simulink model "sensorMCUSlugsMKII_ren"  (Simulink 6.6)
settings: Solver=FixedStepDiscrete  StartTime=0.0  StopTime=10.0  FixedStep=0.01  RelTol=1e-3
InitFcn:
  | mcuInit
values from neighbouring files (symbols this model uses):
  accBiasRateLimit = 2*(.014844)/300*apSampleTime    [mcuInit.m]
  accelXCutTemp = 350.0    (= 350)    [mcuInit.m]
  axTGain1 = -0.0332796    [mcuInit.m]
  axTGain2 = 0.0543519    [mcuInit.m]
  axTMean1 = 68.41    [mcuInit.m]
  axTMean2 = 500.7    [mcuInit.m]
  barAdjust = -6    [mcuInit.m]
  baroCutoff = 0.38/(2*pi)    (= 0.0604788783749)    [mcuInit.m]
  baroCutTemp = -50.0    (= -50)    [mcuInit.m]
  baroOffset = P(2)    [mcuInit.m]
  baroScale = P(1)    [mcuInit.m]
  barTGain1 = -0.0102663    [mcuInit.m]
  barTGain2 = 0.0207608    [mcuInit.m]
  barTMean1 = -161.3    [mcuInit.m]
  barTMean2 = 347.23    [mcuInit.m]
  baseTemp = 288.215    [mcuInit.m]
  cubeAccelGain = (2.522e-3)*9.815    (= 0.02475343)    [mcuInit.m]
  cubeGyroGain = .07326*pi/180    (= 0.00127862821001)    [mcuInit.m]
  gyroBiasRateLimit = 2*(.006393)/500*apSampleTime    [mcuInit.m]
  lapseRate = -0.00198122    [mcuInit.m]
  lowRateSensorCutoff = 0.02    [mcuInit.m]
  magMeanTemp = [162.42 162.42 162.42]    [mcuInit.m]
  magOffset = 0    [mcuInit.m]
  magScale = 0.3418    [mcuInit.m]
  magTempK = [.0057 -.0423 .0426]    [mcuInit.m]
  mainSensorCutoff = 10    [mcuInit.m]
  maxDynPressure = 3000    [mcuInit.m]
  pitAdjust = -41    [mcuInit.m]
  pitCutTemp = -130.0    (= -130)    [mcuInit.m]
  pitotOffset = -1083.881038056753    (= -1083.88103806)    [mcuInit.m]
  pitotScale = 1.213292590242    (= 1.21329259024)    [mcuInit.m]
  pitTGain1 = -0.0552923    [mcuInit.m]
  pitTGain2 = -0.0950433    [mcuInit.m]
  pitTMean1 = -202.93    [mcuInit.m]
  pitTMean2 = 293.053    [mcuInit.m]
  powerOffset = P(2)    [mcuInit.m]
  powerScale = P(1)    [mcuInit.m]
  pressureSensorCutoff = 5    [mcuInit.m]
  T = 0.01    [initGPS.m]    (also in mcuInit.m)
  tempOffset = P(2)    [mcuInit.m]
  tempScale = P(1)    [mcuInit.m]
  vzCutoff = 2    [mcuInit.m]
  xCutoff = 10    [mcuInit.m]
  yCutoff = 10    [mcuInit.m]
  zCutoff = 0.2    [mcuInit.m]
undefined symbols (not defined in the file or in its folder): apSampleTime, baseHeight, DiscIntNeverNeededParam, gaind, getCubeData, getGpsMainData, getMag, GS_location, hil_getEuler, hil_getRates, hil_getRawRead, hil_getVned, hil_getXYZ, hilRead, logData, param_acc, param_mag, polesd, protParseDecode, q_quat, sensorMCUInit, spiSend, u1, u2, updateAirData, updateAttitude, updateBias, updateDiagnosticFl, updateDiagnosticSh, updateLoadData, updatePilotConsole, updatePosition, updateRawADCData, updateTimeStamp, Vb_0, y1, zerosd
libraries: dsPICdrivers x45, simulink x13, aerolibutil x4, dspmtrx3 x2, aerolibconvert2 x2
(part 1 of 4)
settings Model: Creator=ASL_Lab  LastModifiedBy=Administrator  BufferReuse=off  ProdHWDeviceType=16-bit Generic
settings OptimizationCC: BlockReduction=off  InlineParams=on  OptimizeBlockIOStorage=off  BufferReuse=off  ExpressionFolding=off  LocalBlockOutputs=off  EfficientFloat2IntCast=on  OptimizeModelRefInitCode=on  LifeSpan=1
settings HardwareCC: ProdBitPerInt=16  ProdEndianess=LittleEndian  ProdWordSize=16  ProdHWDeviceType=16-bit Generic  TargetHWDeviceType=32-bit Generic
settings RTWCC: SystemTargetFile=dspic.tlc  TemplateMakefile=dspic_pic30_gcc.tmf  PostCodeGenCommand=dsPIC_Compile()  Description=Embedded Target for Microchip dsPIC (real-time)  GenerateReport=on  ProcessScript=dspic_make_rtw_hook  CustomHeaderCode="#include \"apDefinitions.h\""  IncludeHyperlinkInReport=on  LaunchReport=on
settings RTWCC: CustomSource=|
  | clib\circBuffer.c
  | clib\sbrk.c
  | clib\gps.c
  | clib\dataLogger.c
  | clib\interProcCommMaster.c
  | clib\conversions.c
  | clib\apUtils.c
  | clib\protDecoder.c
  | clib\DEE.c
  | clib\DEES.s
  | clib\magneto.c
  | clib\adisCube.c
settings CodeAppCC: IgnoreCustomStorageClasses=off
settings STFCustomTargetCC: TargetFcnLib=ansi_tfl_tmw.mat  GenFloatMathFcnCalls=ANSI_C  ModelReferenceCompliant=off  IncludeMdlTerminateFcn=off  CombineOutputUpdateFcns=on  SuppressErrorStatus=on  ERTCustomFileBanners=on  SupportContinuousTime=off  SupportNonInlinedSFcns=off  SystemTargetFile=dspic.tlc
settings ERTTargetCC: TargetFcnLib=ansi_tfl_tmw.mat  GenFloatMathFcnCalls=ANSI_C  ModelReferenceCompliant=off  IncludeMdlTerminateFcn=off  SuppressErrorStatus=on  ModelStepFunctionPrototypeControlCompliant=off  ExtModeMexFile=noextcomm  InlinedParameterPlacement=NonHierarchical  ERTSrcFileBannerTemplate=dsPIC_code_template.cgt  ERTHdrFileBannerTemplate=dsPIC_code_template.cgt  ERTDataSrcFileTemplate=dsPIC_code_template.cgt  ERTDataHdrFileTemplate=dsPIC_code_template.cgt  ERTCustomFileTemplate=dsPIC_main.tlc
settings CustomProperty: DataType=string  Value=C:\PROGRA~1\MATLAB\R2007a\rtw\bin\win32\gmake

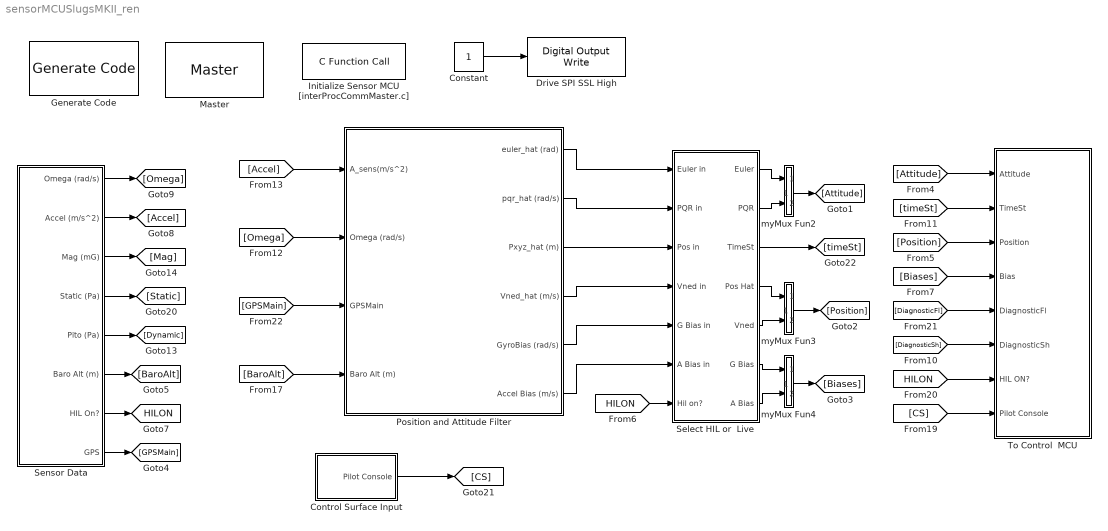
== system sensorMCUSlugsMKII_ren ==
  Constant : Constant  OutDataTypeMode=boolean
  Control Surface Input : Subsystem
  Drive SPI SSL High : dsPICdrivers/Digital I//O/Digital Output Write  Tag=dsPIC_Digital_Output  Priority=5  PORT=B  Pin=[ 2]  Simultaneous=off  OrderingInOutPopup=None
  Generate Code : dsPICdrivers/Simulink Configuration/Generate Code
  Initialize Sensor MCU [interProcCommMaster.c] : dsPICdrivers/OTHERS/C Function Call  Tag=dsPIC_dsPIC_CFunctionCall  fctName='sensorMCUInit'  INPUT_SIZE=1  INPUT1=--  INPUT2=--  INPUT3=--  OUTPUT_SIZE=1  OUTPUT1=--  SampleTime=inf  InputType=[ ]  OutputType=[ ]  FctDeclaration=extern void sensorMCUInit();  FctCall=sensorMCUInit();  OrderingInOutPopup=None
  Master : dsPICdrivers/Master  Tag=dsPIC_MASTER  Priority=1  TimeStepType=Timer1  picType=33fJ256MC710  fcy=40000000  Quartz_33f=12e6  PLLActive_33f=on  fcyDesired_33f=40e6  tmr1="[8  49999  0]"  tmr1Info="Time Step : 0.01  ;   Error : 0%  PR1=49999"  tmr2345="[8  0  0  0  0  0  0  0]"  tmr2345cfg=[-1 -1 -1 -1 -1 -1 -1 -1]  IOautoConf=on  typePort="[ 0   0   0   0   0   0   0   0   0   0   0   0   0   0   9   0   0   0  10   0   0   0   0   0   8   8   8   8   0   0   0   0   0   0   0   0   0   0   0   0   0   0   0   0   0   0   0   0   0   0   9   0   0   0   0   0   0   6   6   6   6   0   0   6   0   0   0   0   0   0   0   0   0   0   0   0   0   0   0   0   0   0   0   0   0   0   0   0   0   0   0   0   0   0   0   0   0   0   0   0   0   0   0   0   0   0   0   0   0   0   0   0 ]"  TRIS="[ 65535  65531  65535  65535  65535  65535  65535 ]"  ADPCFG=4  MasterBusyPort=None  MasterOverloadPort=None  FOSC=External Clock  ClockSwitchMonitor=Both disabled  TempProtection_33f=TEMP_ON  FPBOR=<empty>  PWRT=64ms  MCLR=<empty>  PowerSave=off  OverrideFcy=off  NewFcy=1e6  PR2345="[65535  65535  65535  65535  65535  65535  65535  65535]"
  Position and Attitude Filter : Subsystem
  Select HIL or  Live : Subsystem
  Sensor Data : Subsystem
  To Control  MCU : Subsystem
  myMux Fun2 : Stateflow chart
  myMux Fun3 : Stateflow chart
  myMux Fun4 : Stateflow chart
  tag scope: HILON=global
  wires:
  Constant/1 -> Drive SPI SSL High/1
  myMux Fun2/1(y) -> [Attitude]
  myMux Fun3/1(y) -> [Position]
  myMux Fun4/1(y) -> [Biases]
  Control Surface Input/1(Pilot Console) -> [CS]
  [Position] -> To Control  MCU/3(Position)
  [Biases] -> To Control  MCU/4(Bias)
  [DiagnosticFl] -> To Control  MCU/5(DiagnosticFl)
  [HILON] -> To Control  MCU/7(HIL ON?)
  [CS] -> To Control  MCU/8(Pilot Console)
  [Attitude] -> To Control  MCU/1(Attitude)
  Select HIL or  Live/1(Euler) -> myMux Fun2/1(u1)
  Select HIL or  Live/2(PQR) -> myMux Fun2/2(u2)
  Select HIL or  Live/3(TimeSt) -> [timeSt]
  Select HIL or  Live/4(Pos Hat) -> myMux Fun3/1(u1)
  Select HIL or  Live/5(Vned) -> myMux Fun3/2(u2)
  Select HIL or  Live/6(G Bias) -> myMux Fun4/1(u1)
  Select HIL or  Live/7(A Bias) -> myMux Fun4/2(u2)
  [DiagnosticSh] -> To Control  MCU/6(DiagnosticSh)
  [timeSt] -> To Control  MCU/2(TimeSt)
  Sensor Data/2(Accel (m/s^2)) -> [Accel]
  Sensor Data/1(Omega (rad/s)) -> [Omega]
  Sensor Data/3(Mag (mG)) -> [Mag]
  Sensor Data/4(Static (Pa)) -> [Static]
  Sensor Data/5(Pito (Pa)) -> [Dynamic]
  Sensor Data/6(Baro Alt (m)) -> [BaroAlt]
  Sensor Data/7(HIL On?) -> [HILON]
  Sensor Data/8(GPS) -> [GPSMain]
  [HILON] -> Select HIL or  Live/7(Hil on?)
  [Omega] -> Position and Attitude Filter/2(Omega (rad/s))
  [Accel] -> Position and Attitude Filter/1(A_sens(m/s^2))
  Position and Attitude Filter/1(euler_hat (rad)) -> Select HIL or  Live/1(Euler in)
  Position and Attitude Filter/2(pqr_hat (rad/s)) -> Select HIL or  Live/2(PQR in)
  Position and Attitude Filter/3(Pxyz_hat (m)) -> Select HIL or  Live/3(Pos in)
  Position and Attitude Filter/4(Vned_hat (m/s)) -> Select HIL or  Live/4(Vned in)
  Position and Attitude Filter/5(GyroBias (rad/s)) -> Select HIL or  Live/5(G Bias in)
  Position and Attitude Filter/6(Accel Bias (m/s)) -> Select HIL or  Live/6(A Bias in)
  [GPSMain] -> Position and Attitude Filter/3(GPSMain)
  [BaroAlt] -> Position and Attitude Filter/4(Baro Alt (m))

== system sensorMCUSlugsMKII_ren/Control Surface Input ==
  Input Capture : dsPICdrivers/Peripheral I//O/Input Capture  Tag=dsPIC_PWM_IC  Priority=5  IntPriority=6  Channel=[ 2 3 4 5 8]  Channel_UP_Down_Periode="[1  1  1  1  1]"  MaxChannel="[0.0025      0.0025      0.0025      0.0025      0.0025]"  SafeMarge="[10  10  10  10  10]"  MaxName=' IC2max , IC3max , IC4max , IC5max , IC8max '  Precision="[13.7469      13.7469      13.7469      13.7469      13.7469]"  Timer="[2  2  2  2  2]"  ChangeDetected="[0  0  0  0  0]"  ChangeDetectedPortRef=3  SampleTime=.01  Status=OK
  myMux Fun5 : Stateflow chart
  Pilot Console : Outport
  wires:
  myMux Fun5/1(y) -> Pilot Console/1
  Input Capture/1 -> myMux Fun5/1(u1)
  Input Capture/2 -> myMux Fun5/2(u2)
  Input Capture/3 -> myMux Fun5/3(u3)
  Input Capture/4 -> myMux Fun5/4(u4)
  Input Capture/5 -> myMux Fun5/5(u5)

== system sensorMCUSlugsMKII_ren/Position and Attitude Filter ==
  A_sens(m/s^2) : Inport
  Omega (rad/s) : Inport  Port=2
  GPSMain : Inport  Port=3
  Baro Alt (m) : Inport  Port=4
  Attitude Complimentary Filter COG : Subsystem
  COG.SOG2V : Subsystem
  Compute GS Location : Subsystem
  Constant : Constant  Value=GS_location  OutDataTypeMode=single
  Demux : Demux  Outputs=5
  GPS Update : Subsystem  mask{T=0.01}
      mask prompts: T "Sample Time"
  Geod2LTP1 : Subsystem
      mask Description:
      | This block provides transformation of the Geodetic coordinates
      | to the LTP coorinate system. The block uses two consecutive transformations
      | (Geodetic -> ECEF ->LTP).
      | Geodetic coordinates of the LTP origin should also be predetermined.
      mask Help: Oops!
      mask Display: plot(0,0,100,100,[45,40,35,40,40],[85,95,85,95,40],[85,95,85,95,40],[35,40,45,40,40],[60,40,10,20,10,14],[70,40,10,13,10,20],[56,45],[70,70],[60,60],[50,60],[60,60],[30,40],[50,60],[20,20],[30,40],[20,20],[45,55],[35,25],[75,65],[35,25])
  Position Filter : Subsystem
  "[1 1 -1]" : Gain  Gain=[1 1 -1]
  euler_hat (rad) : Outport
  pqr_hat (rad/s) : Outport  Port=2
  Pxyz_hat (m) : Outport  Port=3
  Vned_hat (m/s) : Outport  Port=4
  GyroBias (rad/s) : Outport  Port=5
  Accel Bias (m/s) : Outport  Port=6
  wires:
  Position Filter/1(Vxyd_hat) -> Vned_hat (m/s)/1, Attitude Complimentary Filter COG/4(Vxyd_hat)
  Position Filter/2(Pxyd_hat) -> Pxyz_hat (m)/1
  Position Filter/3(acc_bias) -> Accel Bias (m/s)/1, Attitude Complimentary Filter COG/5(acc_bias)
  Geod2LTP1/1("NEU, m") -> GPS Update/1(XYZ), "[1 1 -1]"/1
  Attitude Complimentary Filter COG/4(RL2B) -> Position Filter/3(RLT2B)
  Attitude Complimentary Filter COG/1(euler_hat) -> euler_hat (rad)/1
  Attitude Complimentary Filter COG/2(pqr_hat) -> pqr_hat (rad/s)/1
  Attitude Complimentary Filter COG/3(Gyro Bias) -> GyroBias (rad/s)/1
  GPSMain/1 -> Demux/1
  Constant/1 -> Compute GS Location/1(GS Location)
  Demux/1 -> Geod2LTP1/3("Lat, deg(GPS)")
  Demux/2 -> Geod2LTP1/4("Lon, deg(GPS)")
  Demux/3 -> Geod2LTP1/5(Hight,m(GPS))
  Compute GS Location/2(R_in) -> Geod2LTP1/2(GS ECEF)
  Compute GS Location/1("Lat, Lon") -> Geod2LTP1/1(GS Lat,Lon)
  GPS Update/1(Update?) -> Position Filter/6(NewGPS)
  A_sens(m/s^2)/1 -> Attitude Complimentary Filter COG/1(A_sens)
  Omega (rad/s)/1 -> Attitude Complimentary Filter COG/3(Gyros)
  "[1 1 -1]"/1 -> Position Filter/2(GPS_XYD)
  [XY_Orient] -> Attitude Complimentary Filter COG/2(XY Orient)
  Baro Alt (m)/1 -> Position Filter/1(Baro Alt)
  Demux/4 -> COG.SOG2V/1(COG_D)
  Demux/5 -> COG.SOG2V/2(SOG), Position Filter/7(SOG)
  COG.SOG2V/1(Vnorth) -> Position Filter/4(Vnorth)
  COG.SOG2V/2(Veast) -> Position Filter/5(Veast)
  COG.SOG2V/3(XY Orient) -> [XY_Orient]

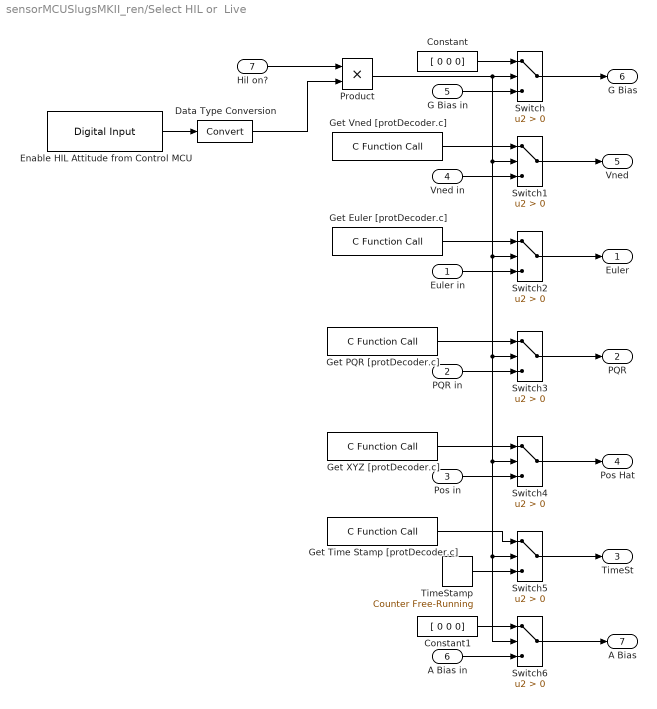
== system sensorMCUSlugsMKII_ren/Select HIL or  Live ==
  Euler in : Inport
  PQR in : Inport  Port=2
  Pos in : Inport  Port=3
  Vned in : Inport  Port=4
  G Bias in : Inport  Port=5
  A Bias in : Inport  Port=6
  Hil on? : Inport  Port=7
  Constant : Constant  Value=[ 0 0 0]  OutDataTypeMode=single
  Constant1 : Constant  Value=[ 0 0 0]  OutDataTypeMode=single
  Data Type Conversion : DataTypeConversion  OutDataTypeMode=uint8
  Enable HIL Attitude from Control MCU : dsPICdrivers/Digital I//O/Digital Input  Tag=dsPIC_Digital_Input  PORT=A  Pin=[14]  SampleTime=.01  OrderingInOutPopup=None
  Get Euler [protDecoder.c] : dsPICdrivers/OTHERS/C Function Call  Tag=dsPIC_dsPIC_CFunctionCall  fctName='hil_getEuler'  INPUT_SIZE=1  INPUT1=--  INPUT2=--  INPUT3=--  OUTPUT_SIZE=3  OUTPUT1=real32  SampleTime=.01  InputType=[ ]  OutputType=[ 7 ]  FctDeclaration=extern void hil_getEuler(real32_T* y1);  FctCall=hil_getEuler(*%y1);  OrderingInOutPopup=None
  Get PQR [protDecoder.c] : dsPICdrivers/OTHERS/C Function Call  Tag=dsPIC_dsPIC_CFunctionCall  fctName='hil_getRates'  INPUT_SIZE=1  INPUT1=--  INPUT2=--  INPUT3=--  OUTPUT_SIZE=3  OUTPUT1=real32  SampleTime=.01  InputType=[ ]  OutputType=[ 7 ]  FctDeclaration=extern void hil_getRates(real32_T* y1);  FctCall=hil_getRates(*%y1);  OrderingInOutPopup=None
  Get Time Stamp [protDecoder.c] : dsPICdrivers/OTHERS/C Function Call  Tag=dsPIC_dsPIC_CFunctionCall  fctName='hil_getTs'  INPUT_SIZE=1  INPUT1=--  INPUT2=--  INPUT3=--  OUTPUT_SIZE=1  OUTPUT1=uint16  SampleTime=.01  InputType=[ ]  OutputType=[ 4 ]  FctDeclaration=extern uint16_T hil_getTs();  FctCall=%y1 = hil_getTs();  OrderingInOutPopup=None
  Get Vned [protDecoder.c] : dsPICdrivers/OTHERS/C Function Call  Tag=dsPIC_dsPIC_CFunctionCall  fctName='hil_getVned'  INPUT_SIZE=1  INPUT1=--  INPUT2=--  INPUT3=--  OUTPUT_SIZE=3  OUTPUT1=real32  SampleTime=.01  InputType=[ ]  OutputType=[ 7 ]  FctDeclaration=extern void hil_getVned(real32_T* y1);  FctCall=hil_getVned(*%y1);  OrderingInOutPopup=None
  Get XYZ [protDecoder.c] : dsPICdrivers/OTHERS/C Function Call  Tag=dsPIC_dsPIC_CFunctionCall  fctName='hil_getXYZ'  INPUT_SIZE=1  INPUT1=--  INPUT2=--  INPUT3=--  OUTPUT_SIZE=3  OUTPUT1=real32  SampleTime=.01  InputType=[ ]  OutputType=[ 7 ]  FctDeclaration=extern void hil_getXYZ(real32_T* y1);  FctCall=hil_getXYZ(*%y1);  OrderingInOutPopup=None
  Product : Product  OutDataTypeMode=uint8  RndMeth=Zero
  Switch{,1..6} (7 alike) : Switch  Criteria=u2 > Threshold
  TimeStamp : simulink/Sources/Counter Free-Running  SystemSampleTime=-1  NumBits=16  tsamp=.01
  Euler : Outport
  PQR : Outport  Port=2
  TimeSt : Outport  Port=3
  Pos Hat : Outport  Port=4
  Vned : Outport  Port=5
  G Bias : Outport  Port=6
  A Bias : Outport  Port=7
  wires:
  Switch/1 -> G Bias/1
  Constant/1 -> Switch/1
  Product/1 -> Switch/2, Switch1/2, Switch2/2, Switch3/2, Switch4/2, Switch5/2, Switch6/2
  G Bias in/1 -> Switch/3
  Switch1/1 -> Vned/1
  Get Vned [protDecoder.c]/1 -> Switch1/1
  Vned in/1 -> Switch1/3
  Get Euler [protDecoder.c]/1 -> Switch2/1
  Euler in/1 -> Switch2/3
  Switch2/1 -> Euler/1
  Get PQR [protDecoder.c]/1 -> Switch3/1
  PQR in/1 -> Switch3/3
  Switch3/1 -> PQR/1
  Get XYZ [protDecoder.c]/1 -> Switch4/1
  Pos in/1 -> Switch4/3
  Switch4/1 -> Pos Hat/1
  TimeStamp/1 -> Switch5/3
  Get Time Stamp [protDecoder.c]/1 -> Switch5/1
  Enable HIL Attitude from Control MCU/1 -> Data Type Conversion/1
  Hil on?/1 -> Product/1
  Data Type Conversion/1 -> Product/2
  Switch5/1 -> TimeSt/1
  Switch6/1 -> A Bias/1
  Constant1/1 -> Switch6/1
  A Bias in/1 -> Switch6/3

== system sensorMCUSlugsMKII_ren/Sensor Data ==
  Data Type Conversion : DataTypeConversion  OutDataTypeMode=uint8  SampleTime=0.01
  Enable HIL from  Control MCU : dsPICdrivers/Digital I//O/Digital Input  Tag=dsPIC_Digital_Input  PORT=D  Pin=[2]  SampleTime=.01  OrderingInOutPopup=None
  Raw HIL  Readings : Subsystem
  Sensor Suite : Subsystem
  Omega (rad/s) : Outport
  Accel (m/s^2) : Outport  Port=2
  Mag (mG) : Outport  Port=3
  Static (Pa) : Outport  Port=4
  Pito (Pa) : Outport  Port=5
  Baro Alt (m) : Outport  Port=6
  HIL On? : Outport  Port=7
  GPS : Outport  Port=8
  wires:
  Raw HIL  Readings/1(Raw Msg) -> Sensor Suite/2(Raw HIL)
  Enable HIL from  Control MCU/1 -> Raw HIL  Readings/Enable, Sensor Suite/1(D2), Data Type Conversion/1
  Data Type Conversion/1 -> HIL On?/1
  Sensor Suite/1(Omega (rad/s)) -> Omega (rad/s)/1
  Sensor Suite/2(Accel (m/s^2)) -> Accel (m/s^2)/1
  Sensor Suite/3(Mag (mG)) -> Mag (mG)/1
  Sensor Suite/4(Static (Pa)) -> Static (Pa)/1
  Sensor Suite/5(Pitot (Pa)) -> Pito (Pa)/1
  Sensor Suite/6(Baro Alt (m)) -> Baro Alt (m)/1
  Sensor Suite/7(GPS) -> GPS/1

== system sensorMCUSlugsMKII_ren/To Control  MCU ==
  Attitude : Inport
  TimeSt : Inport  Port=2
  Position : Inport  Port=3
  Bias : Inport  Port=4
  DiagnosticFl : Inport  Port=5
  DiagnosticSh : Inport  Port=6
  HIL ON? : Inport  Port=7
  Pilot Console : Inport  Port=8
  IPC Data : Subsystem
  Send Debug  Data to Serial Port and Prepare for SPI [dataLogger.c] : dsPICdrivers/OTHERS/C Function Call  Tag=dsPIC_dsPIC_CFunctionCall  fctName='logData'  INPUT_SIZE=1  INPUT1=uint8  INPUT2=--  INPUT3=--  OUTPUT_SIZE=104  OUTPUT1=uint8  SampleTime=-1  InputType=[ 2 ]  OutputType=[ 2 ]  FctDeclaration=extern void logData(uint8_T u1,uint8_T* y1);  FctCall=logData(%u1, *%y1);  OrderingInOutPopup=Input
  Update Biases [dataLogger.c] : dsPICdrivers/OTHERS/C Function Call  Tag=dsPIC_dsPIC_CFunctionCall  fctName='updateBias'  INPUT_SIZE=6  INPUT1=real32  INPUT2=--  INPUT3=--  OUTPUT_SIZE=1  OUTPUT1=--  SampleTime=.01  InputType=[ 7 ]  OutputType=[ ]  FctDeclaration=extern void updateBias(real32_T* u1);  FctCall=updateBias(*%u1);  OrderingInOutPopup=Input & Output
  Update Diagnostic Float [dataLogger.c] : dsPICdrivers/OTHERS/C Function Call  Tag=dsPIC_dsPIC_CFunctionCall  fctName='updateDiagnosticFl'  INPUT_SIZE=3  INPUT1=real32  INPUT2=--  INPUT3=--  OUTPUT_SIZE=1  OUTPUT1=--  SampleTime=.01  InputType=[ 7 ]  OutputType=[ ]  FctDeclaration=extern void updateDiagnosticFl(real32_T* u1);  FctCall=updateDiagnosticFl(*%u1);  OrderingInOutPopup=Input & Output
  Update Diagnostic Short [dataLogger.c] : dsPICdrivers/OTHERS/C Function Call  Tag=dsPIC_dsPIC_CFunctionCall  fctName='updateDiagnosticSh'  INPUT_SIZE=3  INPUT1=int16  INPUT2=--  INPUT3=--  OUTPUT_SIZE=1  OUTPUT1=--  SampleTime=.01  InputType=[ 3 ]  OutputType=[ ]  FctDeclaration=extern void updateDiagnosticSh(int16_T* u1);  FctCall=updateDiagnosticSh(*%u1);  OrderingInOutPopup=Input & Output
  Update Euler and PQR [dataLogger.c] : dsPICdrivers/OTHERS/C Function Call  Tag=dsPIC_dsPIC_CFunctionCall  fctName='updateAttitude'  INPUT_SIZE=6  INPUT1=real32  INPUT2=--  INPUT3=--  OUTPUT_SIZE=1  OUTPUT1=--  SampleTime=.01  InputType=[ 7 ]  OutputType=[ ]  FctDeclaration=extern void updateAttitude(real32_T* u1);  FctCall=updateAttitude(*%u1);  OrderingInOutPopup=Output
  Update Pilot Console [dataLogger.c] : dsPICdrivers/OTHERS/C Function Call  Tag=dsPIC_dsPIC_CFunctionCall  fctName='updatePilotConsole'  INPUT_SIZE=5  INPUT1=uint16  INPUT2=--  INPUT3=--  OUTPUT_SIZE=1  OUTPUT1=--  SampleTime=.01  InputType=[ 4 ]  OutputType=[ ]  FctDeclaration=extern void updatePilotConsole(uint16_T* u1);  FctCall=updatePilotConsole(*%u1);  OrderingInOutPopup=Input & Output
  Update XYZ and Vned [dataLogger.c] : dsPICdrivers/OTHERS/C Function Call  Tag=dsPIC_dsPIC_CFunctionCall  fctName='updatePosition'  INPUT_SIZE=6  INPUT1=real32  INPUT2=--  INPUT3=--  OUTPUT_SIZE=1  OUTPUT1=--  SampleTime=.01  InputType=[ 7 ]  OutputType=[ ]  FctDeclaration=extern void updatePosition(real32_T* u1);  FctCall=updatePosition(*%u1);  OrderingInOutPopup=Input & Output
  Update the Time Stamp [dataLogger.c] : dsPICdrivers/OTHERS/C Function Call  Tag=dsPIC_dsPIC_CFunctionCall  fctName='updateTimeStamp'  INPUT_SIZE=1  INPUT1=uint16  INPUT2=--  INPUT3=--  OUTPUT_SIZE=1  OUTPUT1=--  SampleTime=.01  InputType=[ 4 ]  OutputType=[ ]  FctDeclaration=extern void updateTimeStamp(uint16_T u1);  FctCall=updateTimeStamp(%u1);  OrderingInOutPopup=Input & Output
  wires:
  Send Debug  Data to Serial Port and Prepare for SPI [dataLogger.c]/1 -> IPC Data/1(To SPI)
  HIL ON?/1 -> Send Debug  Data to Serial Port and Prepare for SPI [dataLogger.c]/1
  Attitude/1 -> Update Euler and PQR [dataLogger.c]/1
  Update Euler and PQR [dataLogger.c]/1 -> Update the Time Stamp [dataLogger.c]/2
  TimeSt/1 -> Update the Time Stamp [dataLogger.c]/1
  Update the Time Stamp [dataLogger.c]/1 -> Update XYZ and Vned [dataLogger.c]/2
  Position/1 -> Update XYZ and Vned [dataLogger.c]/1
  Update XYZ and Vned [dataLogger.c]/1 -> Update Pilot Console [dataLogger.c]/2
  Pilot Console/1 -> Update Pilot Console [dataLogger.c]/1
  DiagnosticFl/1 -> Update Diagnostic Float [dataLogger.c]/1
  Update Pilot Console [dataLogger.c]/1 -> Update Diagnostic Float [dataLogger.c]/2
  Update Diagnostic Float [dataLogger.c]/1 -> Update Diagnostic Short [dataLogger.c]/2
  DiagnosticSh/1 -> Update Diagnostic Short [dataLogger.c]/1
  Update Biases [dataLogger.c]/1 -> Send Debug  Data to Serial Port and Prepare for SPI [dataLogger.c]/2
  Update Diagnostic Short [dataLogger.c]/1 -> Update Biases [dataLogger.c]/2
  Bias/1 -> Update Biases [dataLogger.c]/1

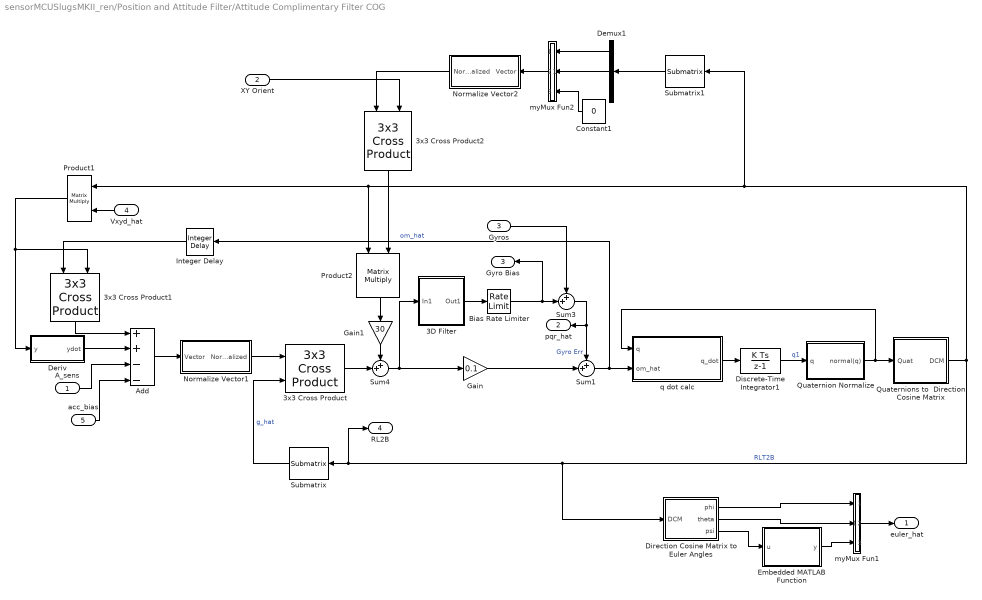
== system sensorMCUSlugsMKII_ren/Position and Attitude Filter/Attitude Complimentary Filter COG ==
  A_sens : Inport  PortDimensions=3
  XY Orient : Inport  Port=2  DataType=single
  Gyros : Inport  Port=3  PortDimensions=3
  Vxyd_hat : Inport  Orientation=left  Port=4  PortDimensions=3
  acc_bias : Inport  Port=5  PortDimensions=3
  3D Filter : Subsystem  AncestorBlock=SLUGS_Library/Singnal Routing & Conditioning/3D Filter  RTWFcnName=TustinFilter3D  mask{zval=[], pval=[0], kval=1, TSample=0.01}
      mask prompts: zval "Zeros"; pval "Poles"; kval "Gains"; TSample "Sample Time"
      settings: RTWFcnNameOpts=User specified  RTWFileNameOpts=Use function name
      mask Display:
      | droots(zval,pval,kval)
      | port_label('input',1,'3D')
  3x3 Cross Product : aerolibutil/3x3 Cross Product  SystemSampleTime=-1
  3x3 Cross Product1 : aerolibutil/3x3 Cross Product  Orientation=down  SystemSampleTime=-1
  3x3 Cross Product2 : aerolibutil/3x3 Cross Product  Orientation=down  SystemSampleTime=-1
  Add : Sum  Inputs=++--  OutScaling=2^-10
  Bias Rate Limiter : RateLimiter  RisingSlewLimit=gyroBiasRateLimit  FallingSlewLimit=-gyroBiasRateLimit  SampleTimeMode=inherited
  Constant1 : Constant  Orientation=left  Value=0  OutDataTypeMode=single
  Demux1 : Demux  Orientation=left  Outputs=3
  "Deriv " : Subsystem
  Direction Cosine Matrix to Euler Angles : Subsystem  AncestorBlock=aerolibtransform2/Direction Cosine Matrix to Euler Angles  mask(DCM2Euler){}
      mask help: Determine an euler orientation (roll, pitch, yaw) from the 3-by-3 direction cosine matrix (DCM). The input DCM transforms vectors from geodetic earth or north-down-east (NED) axes to body axes.
      mask init:
      | aeroicon('aeroblk');
      mask Help: web(asbhelp('directioncosinematrixtoeulerangles'));
      mask Display:
      | port_label('output',1,'\phi','texmode','on')
      | port_label('output',2,'\theta','texmode','on')
      | port_label('output',3,'\psi','texmode','on')
      | port_label('input',1,'DCM_{be}','texmode','on')
  Discrete-Time Integrator1 : DiscreteIntegrator  InitialCondition=q_quat  SampleTime=apSampleTime  LimitOutput=on  UpperSaturationLimit=[1 1 1 1]  LowerSaturationLimit=[-1 -1 -1 -1]  ICPrevOutput=DiscIntNeverNeededParam  ICPrevScaledInput=DiscIntNeverNeededParam
  Embedded MATLAB Function : Stateflow chart
  Gain : Gain  Gain=0.1
  Gain1 : Gain  Orientation=down  Gain=30
  Integer Delay : simulink/Discrete/Integer Delay  Orientation=left  vinit=0.0  samptime=-1  NumDelays=1
  Normalize Vector1 : Subsystem  AncestorBlock=SLUGS_Library/Navigation/Normalize Vector
  Normalize Vector2 : Subsystem  Orientation=left  AncestorBlock=SLUGS_Library/Navigation/Normalize Vector
  Product1 : Product  Orientation=left  Multiplication=Matrix(*)  RndMeth=Zero
  Product2 : Product  Orientation=down  Multiplication=Matrix(*)  RndMeth=Zero
  Quaternion Normalize : Subsystem  AncestorBlock=aerolibutil/Quaternion Normalize  mask(Quaternion Normalize){}
      mask help: Normalize a quaternion.
      mask init:
      | aeroicon('aeroblk');
      mask Help: web(asbhelp);
  Quaternions to  Direction Cosine Matrix : Subsystem  AncestorBlock="aerolibtransform2/Quaternions to  Direction Cosine Matrix"  mask(Quaternion2DCM){}
      mask help: Determine the 3-by-3 direction cosine matrix (DCM) from a 4-by-1 quaternion orientation vector. The output DCM transforms vectors from geodetic earth or north-east-down (NED) axes to body axes.
      mask init:
      | aeroicon('aeroblk');
      mask Help: web(asbhelp('quaternionstodirectioncosinematrix'));
      mask Display:
      | port_label('input',1,'q_n_o_r_m','texmode','on')
      | port_label('output',1,'DCM_{be}','texmode','on')
  Submatrix : dspmtrx3/Submatrix  Orientation=left  RowSpan=Range of rows  RowStartMode=First  RowStartIndex=1  RowEndMode=Last  RowEndIndex=1  ColSpan=One column  ColStartMode=Last  ColStartIndex=1  ColEndMode=Last  ColEndIndex=1
  Submatrix1 : dspmtrx3/Submatrix  Orientation=left  RowSpan=One row  RowStartMode=First  RowStartIndex=1  RowEndMode=Last  RowEndIndex=1  ColSpan=All columns  ColStartMode=Last  ColStartIndex=1  ColEndMode=Last  ColEndIndex=1
  Sum1 : Sum  Inputs=++|
  Sum3 : Sum  Inputs=++|
  Sum4 : Sum  Inputs=++|
  myMux Fun1 : Stateflow chart
  myMux Fun2 : Stateflow chart  Orientation=left
  q dot calc : Stateflow chart
  euler_hat : Outport
  pqr_hat : Outport  Orientation=left  Port=2
  Gyro Bias : Outport  Orientation=left  Port=3
  RL2B : Outport  Port=4
  wires:
  Bias Rate Limiter/1 -> Gyro Bias/1, Sum3/2
  Product2/1 -> Gain1/1
  Gain1/1 -> Sum4/1
  Normalize Vector2/1(Normalized) -> 3x3 Cross Product2/1
  myMux Fun2/1(y) -> Normalize Vector2/1(Vector)
  Constant1/1 -> myMux Fun2/3(u3)
  Demux1/2 -> myMux Fun2/2(u2)
  Demux1/1 -> myMux Fun2/1(u1)
  Submatrix1/1 -> Demux1/1
  Sum1/1 -> q dot calc/2(om_hat), Integer Delay/1  "om_hat"
  q dot calc/1(q_dot) -> Discrete-Time Integrator1/1
  Submatrix/1 -> 3x3 Cross Product/2  "g_hat"
  Sum4/1 -> Gain/1, 3D Filter/1(In1)
  3x3 Cross Product1/1 -> Add/1
  A_sens/1 -> Add/3
  Normalize Vector1/1(Normalized) -> 3x3 Cross Product/1
  3x3 Cross Product/1 -> Sum4/2
  Quaternions to  Direction Cosine Matrix/1(DCM) -> Submatrix1/1, Product2/1, Product1/1, Submatrix/1, RL2B/1, Direction Cosine Matrix to Euler Angles/1(DCM)  "RLT2B"
  Integer Delay/1 -> 3x3 Cross Product1/1
  Discrete-Time Integrator1/1 -> Quaternion Normalize/1(q)  "q1"
  Quaternion Normalize/1(normal(q)) -> Quaternions to  Direction Cosine Matrix/1(Quat), q dot calc/1(q)
  "Deriv "/1(ydot) -> Add/2
  Add/1 -> Normalize Vector1/1(Vector)
  acc_bias/1 -> Add/4
  Product1/1 -> 3x3 Cross Product1/2, "Deriv "/1(y)
  Vxyd_hat/1 -> Product1/2
  Direction Cosine Matrix to Euler Angles/3(psi) -> Embedded MATLAB Function/1(u)
  myMux Fun1/1(y) -> euler_hat/1
  Direction Cosine Matrix to Euler Angles/1(phi) -> myMux Fun1/1(u1)
  Direction Cosine Matrix to Euler Angles/2(theta) -> myMux Fun1/2(u2)
  Embedded MATLAB Function/1(y) -> myMux Fun1/3(u3)
  3D Filter/1(Out1) -> Bias Rate Limiter/1
  Gyros/1 -> Sum3/1
  Gain/1 -> Sum1/2
  Sum3/1 -> Sum1/1, pqr_hat/1  "Gyro Err"
  XY Orient/1 -> 3x3 Cross Product2/2
  3x3 Cross Product2/1 -> Product2/2

== system sensorMCUSlugsMKII_ren/Position and Attitude Filter/COG.SOG2V ==
  COG_D : Inport
  SOG : Inport  Orientation=left  Port=2
  Angle Conversion : aerolibconvert2/Angle Conversion  SystemSampleTime=-1  IU=deg  OU=rad
  Constant : Constant  Value=0  OutDataTypeMode=single
  Product : Product  RndMeth=Zero
  Product1 : Product  RndMeth=Zero
  Subsystem5 : Subsystem  AncestorBlock=SLUGS_Library/Subsystem5
  myMux Fun2 : Stateflow chart
  Vnorth : Outport
  Veast : Outport  Port=2
  XY Orient : Outport  Port=3
  wires:
  Product1/1 -> Vnorth/1
  Product/1 -> Veast/1
  SOG/1 -> Product1/1, Product/2
  Angle Conversion/1 -> Subsystem5/1(u)
  Subsystem5/1(sin(u)) -> Product/1, myMux Fun2/2(u2)
  Subsystem5/2(cos(u)) -> Product1/2, myMux Fun2/1(u1)
  COG_D/1 -> Angle Conversion/1
  Constant/1 -> myMux Fun2/3(u3)
  myMux Fun2/1(y) -> XY Orient/1

== system sensorMCUSlugsMKII_ren/Position and Attitude Filter/Compute GS Location ==
  GS Location : Inport
  Demux : Demux  Outputs=3
  Geod2ECEF1 : Subsystem  mask{Re=6378137, Rp=6356752.3142}
      mask prompts: Re "Enter equatorial radius, m"; Rp "Enter polar radius,m"
  Mux1 : Mux  Inputs=2
  Mux2 : Mux  Inputs=3
  "Lat, Lon" : Outport
  R_in : Outport  Port=2
  wires:
  Geod2ECEF1/3("Ze, m ") -> Mux2/3
  Geod2ECEF1/1("Xe, m ") -> Mux2/1
  Geod2ECEF1/2("Ye, m ") -> Mux2/2
  Demux/1 -> Geod2ECEF1/1("height, m")
  Demux/2 -> Mux1/2, Geod2ECEF1/2("lat, deg")
  Demux/3 -> Mux1/1, Geod2ECEF1/3(lon,deg)
  GS Location/1 -> Demux/1
  Mux1/1 -> "Lat, Lon"/1
  Mux2/1 -> R_in/1  "R_in"

== system sensorMCUSlugsMKII_ren/Position and Attitude Filter/GPS Update ==
  XYZ : Inport
  Data Type Conversion2 : DataTypeConversion  OutDataTypeMode=uint8
  Demux : Demux  Outputs=3
  Detect Change : Subsystem
  Detect Change1 : Subsystem
  Detect Change2 : Subsystem
  Rate Transition : RateTransition  OutPortSampleTime=T
  Saturation1 : Saturate  UpperLimit=1  LowerLimit=0  SampleTime=T
  Sum : Sum  Inputs=3
  Update? : Outport
  wires:
  Demux/1 -> Detect Change/1(Data)
  Demux/2 -> Detect Change1/1(Data)
  Demux/3 -> Detect Change2/1(Data)
  Detect Change/1(change?) -> Sum/1
  Detect Change1/1(change?) -> Sum/2
  Detect Change2/1(change?) -> Sum/3
  Sum/1 -> Saturation1/1
  XYZ/1 -> Rate Transition/1
  Saturation1/1 -> Data Type Conversion2/1
  Rate Transition/1 -> Demux/1
  Data Type Conversion2/1 -> Update?/1

== system sensorMCUSlugsMKII_ren/Position and Attitude Filter/Geod2LTP1 ==
  GS Lat,Lon : Inport
  GS ECEF : Inport  Port=2
  "Lat, deg(GPS)" : Inport  Port=3
  "Lon, deg(GPS)" : Inport  Port=4
  Hight,m(GPS) : Inport  Port=5
  ECEF2LTP (UEN) : Subsystem
      mask Display: plot(0,0,100,100,[45,40,35,40,40],[85,95,85,95,40],[85,95,85,95,40],[35,40,45,40,40],[60,40,10,20,10,14],[70,40,10,13,10,20],[56,45],[70,70],[60,60],[50,60],[60,60],[30,40],[50,60],[20,20],[30,40],[20,20],[45,55],[35,25],[75,65],[35,25])
  Geod2ECEF1 : Subsystem  mask{Re=6378137, Rp=6356752.3142}
      mask prompts: Re "Enter equatorial radius, m"; Rp "Enter polar radius,m"
  Mux : Mux  Inputs=3
  Reshape : Reshape  OutputDimensionality=Column vector (2-D)
  Reshape1 : Reshape
  Sum1 : Sum  Inputs=|+-  OutDataTypeMode=single  SaturateOnIntegerOverflow=on
  UEN 2 NEU : Gain  Gain=[0 0 1;0 1 0;1 0 0]  Multiplication=Matrix(K*u)  OutDataTypeMode=Specify via dialog  OutDataType=float('single')  SaturateOnIntegerOverflow=on
  "NEU, m" : Outport
  wires:
  Reshape1/1 -> "NEU, m"/1
  Reshape/1 -> UEN 2 NEU/1
  Sum1/1 -> ECEF2LTP (UEN)/1(ECEF coordinates)
  Mux/1 -> Sum1/1  "r_mov"
  Hight,m(GPS)/1 -> Geod2ECEF1/1("height, m")
  ECEF2LTP (UEN)/1(Out) -> Reshape/1  "Moving Side"
  GS ECEF/1 -> Sum1/2
  GS Lat,Lon/1 -> ECEF2LTP (UEN)/2("Long, Lat")
  "Lon, deg(GPS)"/1 -> Geod2ECEF1/3(lon,deg)
  "Lat, deg(GPS)"/1 -> Geod2ECEF1/2("lat, deg")
  Geod2ECEF1/2("Ye, m ") -> Mux/2
  Geod2ECEF1/1("Xe, m ") -> Mux/1
  Geod2ECEF1/3("Ze, m ") -> Mux/3
  UEN 2 NEU/1 -> Reshape1/1

== system sensorMCUSlugsMKII_ren/Position and Attitude Filter/Position Filter ==
  Baro Alt : Inport
  GPS_XYD : Inport  Port=2
  RLT2B : Inport  Port=3
  Vnorth : Inport  Port=4
  Veast : Inport  Port=5
  NewGPS : Inport  Port=6
  SOG : Inport  Port=7
  BlendPosVel : Subsystem
  Vxyd_hat : Outport
  Pxyd_hat : Outport  Port=2
  acc_bias : Outport  Port=3
  wires:
  BlendPosVel/3(acc_bias) -> acc_bias/1
  BlendPosVel/1(Vxyd_hat) -> Vxyd_hat/1
  BlendPosVel/2(Pxyd_hat) -> Pxyd_hat/1
  Baro Alt/1 -> BlendPosVel/4(BaroAlt)
  Veast/1 -> BlendPosVel/3(Veast)
  Vnorth/1 -> BlendPosVel/2(Vnorth)
  NewGPS/1 -> BlendPosVel/6(NewGPS)
  RLT2B/1 -> BlendPosVel/5(RLT2B)
  GPS_XYD/1 -> BlendPosVel/1(GPS_NED)
  SOG/1 -> BlendPosVel/7(SOG)

== system sensorMCUSlugsMKII_ren/Sensor Data/Raw HIL  Readings ==
  Enable : EnablePort
  GetRawMsg [protDecoder.c] : dsPICdrivers/OTHERS/C Function Call  Tag=dsPIC_dsPIC_CFunctionCall  fctName='hil_getRawRead'  INPUT_SIZE=1  INPUT1=--  INPUT2=--  INPUT3=--  OUTPUT_SIZE=13  OUTPUT1=int16  SampleTime=0.01  InputType=[ ]  OutputType=[ 3 ]  FctDeclaration=extern void hil_getRawRead(int16_T* y1);  FctCall=hil_getRawRead(*%y1);  OrderingInOutPopup=Input
  Parser/Decoder [protDecoder.c] : dsPICdrivers/OTHERS/C Function Call  Tag=dsPIC_dsPIC_CFunctionCall  fctName='protParseDecode'  INPUT_SIZE=103  INPUT1=uint8  INPUT2=--  INPUT3=--  OUTPUT_SIZE=1  OUTPUT1=--  SampleTime=-1  InputType=[ 2 ]  OutputType=[ ]  FctDeclaration=extern void protParseDecode(uint8_T* u1);  FctCall=protParseDecode(*%u1);  OrderingInOutPopup=Output
  Read Data from HIL3 [dataLogger.c] : dsPICdrivers/OTHERS/C Function Call  Tag=dsPIC_dsPIC_CFunctionCall  fctName='hilRead'  INPUT_SIZE=1  INPUT1=--  INPUT2=--  INPUT3=--  OUTPUT_SIZE=103  OUTPUT1=uint8  SampleTime=0.01  InputType=[ ]  OutputType=[ 2 ]  FctDeclaration=extern void hilRead(uint8_T* y1);  FctCall=hilRead(*%y1);  OrderingInOutPopup=None
  Raw Msg : Outport
  wires:
  GetRawMsg [protDecoder.c]/1 -> Raw Msg/1
  Read Data from HIL3 [dataLogger.c]/1 -> Parser/Decoder [protDecoder.c]/1
  Parser/Decoder [protDecoder.c]/1 -> GetRawMsg [protDecoder.c]/1

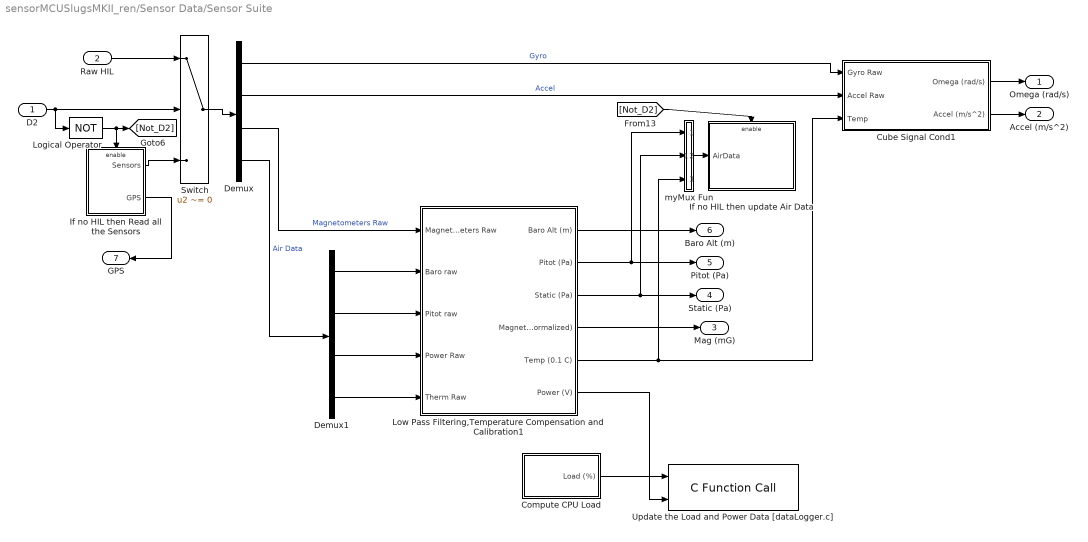
== system sensorMCUSlugsMKII_ren/Sensor Data/Sensor Suite ==
  D2 : Inport
  Raw HIL : Inport  Port=2
  Compute CPU Load : Subsystem
  Cube Signal Cond1 : Subsystem
  Demux : Demux  Outputs=[3 3 3 4]
  Demux1 : Demux
  If no HIL then Read all the Sensors : Subsystem
  If no HIL then update Air Data : Subsystem
  Logical Operator : Logic  Operator=NOT  AllPortsSameDT=off  OutDataTypeMode=Boolean
  Low Pass Filtering,Temperature Compensation and Calibration1 : Subsystem
  Switch : Switch  Criteria=u2 ~= 0  SampleTime=0.01
  Update the Load and Power Data [dataLogger.c] : dsPICdrivers/OTHERS/C Function Call  Tag=dsPIC_dsPIC_CFunctionCall  fctName='updateLoadData'  INPUT_SIZE=1  INPUT1=uint8  INPUT2=uint16  INPUT3=--  OUTPUT_SIZE=1  OUTPUT1=--  SampleTime=.01  InputType=[ 2 4 ]  OutputType=[ ]  FctDeclaration=extern void updateLoadData(uint8_T u1, uint16_T u2);  FctCall=updateLoadData(%u1, %u2);  OrderingInOutPopup=None
  myMux Fun : Stateflow chart
  Omega (rad/s) : Outport
  Accel (m/s^2) : Outport  Port=2
  Mag (mG) : Outport  Port=3
  Static (Pa) : Outport  Port=4
  Pitot (Pa) : Outport  Port=5
  Baro Alt (m) : Outport  Port=6
  GPS : Outport  Orientation=left  Port=7
  wires:
  Switch/1 -> Demux/1
  D2/1 -> Switch/2, Logical Operator/1
  If no HIL then Read all the Sensors/1(Sensors) -> Switch/3
  Logical Operator/1 -> If no HIL then Read all the Sensors/Enable, [Not_D2]
  Raw HIL/1 -> Switch/1
  Low Pass Filtering,Temperature Compensation and Calibration1/1(Baro Alt (m)) -> Baro Alt (m)/1
  Demux/1 -> Cube Signal Cond1/1(Gyro Raw)  "Gyro"
  Demux/4 -> Demux1/1  "Air Data"
  Demux1/1 -> Low Pass Filtering,Temperature Compensation and Calibration1/2(Baro raw)
  Demux1/2 -> Low Pass Filtering,Temperature Compensation and Calibration1/3(Pitot raw)
  Demux1/4 -> Low Pass Filtering,Temperature Compensation and Calibration1/5(Therm Raw)
  Demux/3 -> Low Pass Filtering,Temperature Compensation and Calibration1/1(Magnetometers Raw)  "Magnetometers Raw"
  Demux1/3 -> Low Pass Filtering,Temperature Compensation and Calibration1/4(Power Raw)
  Low Pass Filtering,Temperature Compensation and Calibration1/2(Pitot (Pa)) -> Pitot (Pa)/1, myMux Fun/1(u1)
  Low Pass Filtering,Temperature Compensation and Calibration1/3(Static (Pa)) -> Static (Pa)/1, myMux Fun/2(u2)
  Low Pass Filtering,Temperature Compensation and Calibration1/4(Magnetometer (normalized)) -> Mag (mG)/1
  myMux Fun/1(y) -> If no HIL then update Air Data/1(AirData)
  Low Pass Filtering,Temperature Compensation and Calibration1/5(Temp (0.1 C)) -> myMux Fun/3(u3), Cube Signal Cond1/3(Temp)
  Compute CPU Load/1(Load (%)) -> Update the Load and Power Data [dataLogger.c]/1
  Low Pass Filtering,Temperature Compensation and Calibration1/6(Power (V)) -> Update the Load and Power Data [dataLogger.c]/2
  If no HIL then Read all the Sensors/2(GPS) -> GPS/1
  Demux/2 -> Cube Signal Cond1/2(Accel Raw)  "Accel"
  Cube Signal Cond1/1(Omega (rad/s)) -> Omega (rad/s)/1
  Cube Signal Cond1/2(Accel (m/s^2)) -> Accel (m/s^2)/1
  [Not_D2] -> If no HIL then update Air Data/Enable

== system sensorMCUSlugsMKII_ren/To Control  MCU/IPC Data ==
  To SPI : Inport
  Constant1 : Constant  Value=0  OutDataTypeMode=boolean  SampleTime=.01
  Constant2 : Constant  OutDataTypeMode=boolean
  Drive SSL High : dsPICdrivers/Digital I//O/Digital Output Write  Tag=dsPIC_Digital_Output  Orientation=left  Priority=5  PORT=B  Pin=[ 2]  Simultaneous=off  OrderingInOutPopup=Input
  Drive SSL Low : dsPICdrivers/Digital I//O/Digital Output Write  Tag=dsPIC_Digital_Output  Orientation=left  Priority=5  PORT=B  Pin=[ 2]  Simultaneous=off  OrderingInOutPopup=Output
  Nop : dsPICdrivers/OTHERS/Nop  Tag=dsPIC_Reset  Orientation=up  NbrNop=10
  Nop1 : dsPICdrivers/OTHERS/Nop  Tag=dsPIC_Reset  Orientation=up  NbrNop=10
  Send Data Via SPI [interProcCommMaster.c] : dsPICdrivers/OTHERS/C Function Call  Tag=dsPIC_dsPIC_CFunctionCall  fctName='spiSend'  INPUT_SIZE=104  INPUT1=uint8  INPUT2=--  INPUT3=--  OUTPUT_SIZE=1  OUTPUT1=--  SampleTime=-1  InputType=[ 2 ]  OutputType=[ ]  FctDeclaration=extern void spiSend(uint8_T* u1);  FctCall=spiSend(*%u1);  OrderingInOutPopup=Input & Output
  wires:
  Constant1/1 -> Drive SSL Low/1
  Drive SSL Low/1 -> Nop/1
  Constant2/1 -> Drive SSL High/1
  Send Data Via SPI [interProcCommMaster.c]/1 -> Nop1/1
  To SPI/1 -> Send Data Via SPI [interProcCommMaster.c]/1
  Nop/1 -> Send Data Via SPI [interProcCommMaster.c]/2
  Nop1/1 -> Drive SSL High/2

== system sensorMCUSlugsMKII_ren/Position and Attitude Filter/Attitude Complimentary Filter COG/3D Filter ==
  In1 : Inport
  Data Type Conversion1 : DataTypeConversion  OutDataTypeMode=single
  Data Type Conversion2 : DataTypeConversion  OutDataTypeMode=double
  Demux : Demux  Outputs=3
  Filter1 : Subsystem  mask(DiscretizedZeroPole){Zeros=zval, Poles=pval, Gain=kval, AbsTol=auto, SampleTime=TSample, method=tustin, Wc=1}
      mask prompts: Zeros "Zeros (enter in s-main:)"; Poles "Poles (enter in s-domain:)"; Gain "Gain (enter in s-domain:)"; AbsTol "Absolute tolerance:"; SampleTime "Sample time:"; Wc "Critical Frequency (Hz):"
      mask help: Continuous mask uses c2d to transform parameters onto the Discrete Zero-Pole block inside.
      mask init:
      | st=SampleTime;
      | if length(st)>1
      |     st=SampleTime(1);
      | end
      | if(st>0)
      |     [zerosd,polesd,gaind] = sldiscutil('disczpk', {st,method,Wc,Zeros,Poles,Gain});
      | end	
      | s = get_param(gcb,'maskvalues');
      | zeross = s{1};
      | poless = s{2};
      | gainss = s{3};
      | %zerosc = eval(zeross);
      | %polesc = eval(poless);
      | %gainsc = eval(gainss);
      | sldiscutil('initzpkmask', st);
      | if(st==0)
      | set_param([gcb '/Zero Pole'], 'AbsoluteTolerance', AbsTol);
      | end
      mask StyleString: edit,edit,edit,edit,edit,popup(zoh|foh|tustin|prewarp|matched),edit
      mask CallbackString: |||||hidecrit|
      mask Display:
      | droots(zeross,poless,gainss)
      | text( 0.5, 1.0, method, 'verticalAlignment','top')
  Filter2 : Subsystem  mask(DiscretizedZeroPole){Zeros=zval, Poles=pval, Gain=kval, AbsTol=auto, SampleTime=TSample, method=tustin, Wc=1}
      mask prompts: Zeros "Zeros (enter in s-main:)"; Poles "Poles (enter in s-domain:)"; Gain "Gain (enter in s-domain:)"; AbsTol "Absolute tolerance:"; SampleTime "Sample time:"; Wc "Critical Frequency (Hz):"
      mask help: Continuous mask uses c2d to transform parameters onto the Discrete Zero-Pole block inside.
      mask init: same as sensorMCUSlugsMKII_ren/Position and Attitude Filter/Attitude Complimentary Filter COG/3D Filter/Filter1
      mask StyleString: edit,edit,edit,edit,edit,popup(zoh|foh|tustin|prewarp|matched),edit
      mask CallbackString: |||||hidecrit|
      mask Display:
      | droots(zeross,poless,gainss)
      | text( 0.5, 1.0, method, 'verticalAlignment','top')
  Filter3 : Subsystem  mask(DiscretizedZeroPole){Zeros=zval, Poles=pval, Gain=kval, AbsTol=auto, SampleTime=TSample, method=tustin, Wc=1}
      mask prompts: Zeros "Zeros (enter in s-main:)"; Poles "Poles (enter in s-domain:)"; Gain "Gain (enter in s-domain:)"; AbsTol "Absolute tolerance:"; SampleTime "Sample time:"; Wc "Critical Frequency (Hz):"
      mask help: Continuous mask uses c2d to transform parameters onto the Discrete Zero-Pole block inside.
      mask init: same as sensorMCUSlugsMKII_ren/Position and Attitude Filter/Attitude Complimentary Filter COG/3D Filter/Filter1
      mask StyleString: edit,edit,edit,edit,edit,popup(zoh|foh|tustin|prewarp|matched),edit
      mask CallbackString: |||||hidecrit|
      mask Display:
      | droots(zeross,poless,gainss)
      | text( 0.5, 1.0, method, 'verticalAlignment','top')
  myMux Fun1 : Stateflow chart
  Out1 : Outport
  wires:
  myMux Fun1/1(y) -> Data Type Conversion1/1
  In1/1 -> Data Type Conversion2/1
  Filter3/1(Out1) -> myMux Fun1/3(u3)
  Filter2/1(Out1) -> myMux Fun1/2(u2)
  Filter1/1(Out1) -> myMux Fun1/1(u1)
  Demux/3 -> Filter3/1(In1)
  Demux/2 -> Filter2/1(In1)
  Demux/1 -> Filter1/1(In1)
  Data Type Conversion2/1 -> Demux/1
  Data Type Conversion1/1 -> Out1/1

== system sensorMCUSlugsMKII_ren/Position and Attitude Filter/Attitude Complimentary Filter COG/Deriv  ==
  y : Inport
  Gain2 : Gain  Gain=[ 1/(5*apSampleTime) ]
  Integer Delay1 : simulink/Discrete/Integer Delay  vinit=Vb_0(1)  samptime=apSampleTime  NumDelays=5
  Sum5 : Sum  Inputs=-+|
  ydot : Outport
  wires:
  Sum5/1 -> Gain2/1
  Integer Delay1/1 -> Sum5/1
  y/1 -> Sum5/2, Integer Delay1/1
  Gain2/1 -> ydot/1

== system sensorMCUSlugsMKII_ren/Position and Attitude Filter/Attitude Complimentary Filter COG/Direction Cosine Matrix to Euler Angles ==
  DCM : Inport  PortDimensions=[3,3]
  "Reshape 3x3 -> 9" : Reshape  OutputDimensions=[9, 1]
  Subsystem1 : Subsystem  AncestorBlock=SLUGS_Library/Subsystem4
  Subsystem2 : Subsystem  AncestorBlock=SLUGS_Library/Subsystem4
  Subsystem3 : Subsystem  AncestorBlock=SLUGS_Library/Subsystem6
  cos(phi)cos(theta) : Subsystem
  cos(psi)cos(theta) : Subsystem
  sin(phi)cos(theta) : Subsystem
  sin(psi)cos(theta) : Subsystem
  sin(theta) : Subsystem
  phi : Outport  PortDimensions=1  InitialOutput=0
  theta : Outport  Port=2  PortDimensions=1  InitialOutput=0
  psi : Outport  Port=3  PortDimensions=1  InitialOutput=0
  wires:
  DCM/1 -> "Reshape 3x3 -> 9"/1
  "Reshape 3x3 -> 9"/1 -> sin(theta)/1(DCM), cos(phi)cos(theta)/1(DCM), sin(phi)cos(theta)/1(DCM), cos(psi)cos(theta)/1(DCM), sin(psi)cos(theta)/1(DCM)
  sin(theta)/1(sin(theta)) -> Subsystem3/1(x)
  sin(phi)cos(theta)/1(sin(phi)cos(theta)) -> Subsystem2/1(u)
  cos(phi)cos(theta)/1(cos(phi)cos(theta)) -> Subsystem2/2(v)
  sin(psi)cos(theta)/1(sin(psi)cos(theta)) -> Subsystem1/1(u)
  cos(psi)cos(theta)/1(cos(psi)cos(theta)) -> Subsystem1/2(v)
  Subsystem2/1(atan2(x,y)) -> phi/1  "phi"
  Subsystem3/1(asin(x)) -> theta/1  "theta"
  Subsystem1/1(atan2(x,y)) -> psi/1  "psi"

== system sensorMCUSlugsMKII_ren/Position and Attitude Filter/Attitude Complimentary Filter COG/Normalize Vector1 ==
  Vector : Inport
  Divide : Product  Inputs=*/  OutScaling=2^-10
  Norm : Subsystem  AncestorBlock=SLUGS_Library/Navigation/Norm
  Zero Bound : Saturate  UpperLimit=inf  LowerLimit=0.001
  Normalized : Outport
  wires:
  Divide/1 -> Normalized/1
  Zero Bound/1 -> Divide/2
  Norm/1(Norm) -> Zero Bound/1
  Vector/1 -> Divide/1, Norm/1(Vector)

== system sensorMCUSlugsMKII_ren/Position and Attitude Filter/Attitude Complimentary Filter COG/Normalize Vector2 ==
  Vector : Inport
  Divide : Product  Inputs=*/  OutScaling=2^-10
  Norm : Subsystem  AncestorBlock=SLUGS_Library/Navigation/Norm
  Zero Bound : Saturate  UpperLimit=inf  LowerLimit=0.001
  Normalized : Outport
  wires:
  Vector/1 -> Norm/1(Vector), Divide/1
  Norm/1(Norm) -> Zero Bound/1
  Zero Bound/1 -> Divide/2
  Divide/1 -> Normalized/1

== system sensorMCUSlugsMKII_ren/Position and Attitude Filter/Attitude Complimentary Filter COG/Quaternion Normalize ==
  q : Inport
  Demux : Demux
  Mux : Mux
  Product{,1..3} (4 alike) : Product  Inputs=*/  OutScaling=2^-10
  Quaternion Modulus : Subsystem  AncestorBlock=aerolibutil/Quaternion Modulus  mask(Quaternion Modulus){}
      mask help: Calculate the modulus of a quaternion.
      mask init:
      | aeroicon('aeroblk');
      mask Help: web(asbhelp);
  normal(q) : Outport
  wires:
  Product3/1 -> Mux/4
  Product2/1 -> Mux/3
  Product1/1 -> Mux/2
  Product/1 -> Mux/1
  Quaternion Modulus/1(|q|) -> Product3/2, Product2/2, Product/2, Product1/2
  q/1 -> Quaternion Modulus/1(q), Demux/1
  Mux/1 -> normal(q)/1
  Demux/1 -> Product/1
  Demux/2 -> Product1/1
  Demux/3 -> Product2/1
  Demux/4 -> Product3/1

== system sensorMCUSlugsMKII_ren/Position and Attitude Filter/Attitude Complimentary Filter COG/Quaternions to  Direction Cosine Matrix ==
  Quat : Inport  PortDimensions=4
  A11 : Subsystem
  A12 : Subsystem
  A13 : Subsystem
  A21 : Subsystem
  A22 : Subsystem
  A23 : Subsystem
  A31 : Subsystem
  A32 : Subsystem
  A33 : Subsystem
  Create Transformation Matrix : Subsystem  AncestorBlock=aerolibutil/Create 3x3 Matrix  mask(Create 3x3 Matrix){}
      mask help:
      | Create a 3-by-3 matrix from nine input values. Each input corresponds to an element of the matrix.
      |
      | For example, the input labeled A21 is the entry in the second row and first column of the matrix.
      mask init:
      | aeroicon('aeroblk');
      mask Help: web(asbhelp);
      mask Display:
      | port_label('input',1,'A_{11}','texmode','on');
      | port_label('input',2,'A_{12}','texmode','on');
      | port_label('input',3,'A_{13}','texmode','on');
      | port_label('input',4,'A_{21}','texmode','on');
      | port_label('input',5,'A_{22}','texmode','on');
      | port_label('input',6,'A_{23}','texmode','on');
      | port_label('input',7,'A_{31}','texmode','on');
      | port_label('input',8,'A_{32}','texmode','on');
      | port_label('input',9,'A_{33}','texmode','on');
      | port_label('output',1,'A','texmode','on');
  DCM : Outport  PortDimensions=[3,3]  InitialOutput=0
  wires:
  A12/1(A12) -> Create Transformation Matrix/2(M12)
  A22/1(A22) -> Create Transformation Matrix/5(M22)
  Quat/1 -> A11/1(normal(q)), A12/1(normal(q)), A13/1(normal(q)), A21/1(normal(q)), A22/1(normal(q)), A23/1(normal(q)), A31/1(normal(q)), A32/1(normal(q)), A33/1(normal(q))
  A33/1(A33) -> Create Transformation Matrix/9(M33)
  A23/1(A23) -> Create Transformation Matrix/6(M23)
  A13/1(A13) -> Create Transformation Matrix/3(M13)
  A32/1(A32) -> Create Transformation Matrix/8(M32)
  A31/1(A31) -> Create Transformation Matrix/7(M31)
  A21/1(A21) -> Create Transformation Matrix/4(M21)
  A11/1(A11) -> Create Transformation Matrix/1(M11)
  Create Transformation Matrix/1(Matrix) -> DCM/1

== system sensorMCUSlugsMKII_ren/Position and Attitude Filter/COG.SOG2V/Subsystem5 ==
  u : Inport
  C Function Call : dsPICdrivers/OTHERS/C Function Call  Tag=dsPIC_dsPIC_CFunctionCall  fctName='mySin'  INPUT_SIZE=1  INPUT1=real32  INPUT2=--  INPUT3=--  OUTPUT_SIZE=1  OUTPUT1=real32  SampleTime=-1  InputType=[ 7 ]  OutputType=[ 7 ]  FctDeclaration=extern real32_T mySin(real32_T u1);  FctCall=%y1 = mySin(%u1);  OrderingInOutPopup=None
  C Function Call1 : dsPICdrivers/OTHERS/C Function Call  Tag=dsPIC_dsPIC_CFunctionCall  fctName='myCos'  INPUT_SIZE=1  INPUT1=real32  INPUT2=--  INPUT3=--  OUTPUT_SIZE=1  OUTPUT1=real32  SampleTime=-1  InputType=[ 7 ]  OutputType=[ 7 ]  FctDeclaration=extern real32_T myCos(real32_T u1);  FctCall=%y1 = myCos(%u1);  OrderingInOutPopup=None
  sin(u) : Outport
  cos(u) : Outport  Port=2
  wires:
  u/1 -> C Function Call/1, C Function Call1/1
  C Function Call/1 -> sin(u)/1
  C Function Call1/1 -> cos(u)/1
